simulink model "PardoSplitLabModel"  (R2024b)
settings: Solver=VariableStepAuto  StartTime=0.0  StopTime=10.0  RelTol=1e-3
libraries: simulink x8
settings Model: Creator=ferbe  LastModifiedBy=ferbe

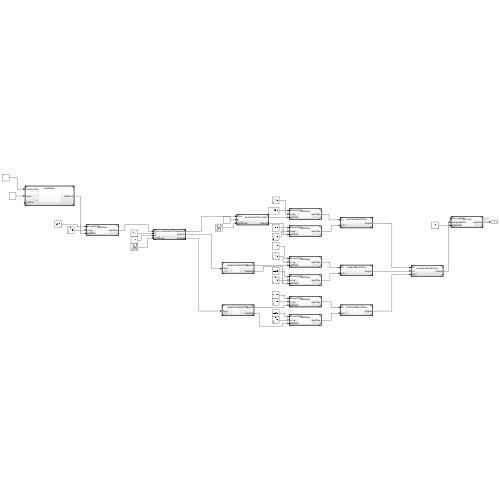
[thumbnail: Simulink's stored preview of the top-level diagram]
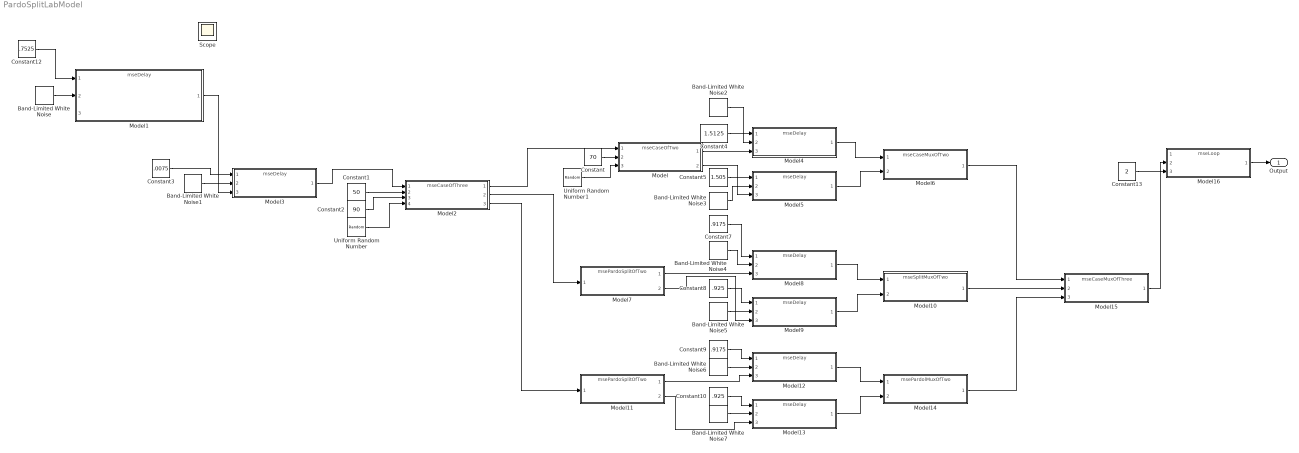
== system PardoSplitLabModel ==
  Band-Limited White Noise{,1..7} (8 alike) : simulink/Sources/Band-Limited White Noise  Cov=[0.1]  Ts=0.1  seed=[23341]
  Constant : Constant  Value=70
  Constant1 : Constant  Value=50
  Constant10 : Constant  Value=.925
  Constant12 : Constant  Value=.7525
  Constant13 : Constant  Value=2
  Constant2 : Constant  Value=90
  Constant3 : Constant  Value=.0075
  Constant4 : Constant  Value=1.5125
  Constant5 : Constant  Value=1.505
  Constant7 : Constant  Value=.9175
  Constant8 : Constant  Value=.925
  Constant9 : Constant  Value=.9175
  Model : ModelReference  ModelNameDialog=mseCaseOfTwo.slx  SimulationMode=Normal  ModelReferenceVersion=3.9
  Model{1,3..5,8..9,12..13} (8 alike) : ModelReference  ModelNameDialog=mseDelay.slx  SimulationMode=Normal  ModelReferenceVersion=3.3
  Model10 : ModelReference  ModelNameDialog=mseSplitMuxOfTwo.slx  SimulationMode=Normal  ModelReferenceVersion=3.2
  Model11 : ModelReference  ModelNameDialog=msePardoSplitOfTwo.slx  SimulationMode=Normal  ModelReferenceVersion=3.2
  Model14 : ModelReference  ModelNameDialog=msePardolMuxOfTwo.slx  SimulationMode=Normal  ModelReferenceVersion=3.3
  Model15 : ModelReference  ModelNameDialog=mseCaseMuxOfThree.slx  SimulationMode=Normal  ModelReferenceVersion=3.1
  Model16 : ModelReference  ModelNameDialog=mseLoop.slx  SimulationMode=Normal  ModelReferenceVersion=3.1
  Model2 : ModelReference  ModelNameDialog=mseCaseOfThree.slx  SimulationMode=Normal  ModelReferenceVersion=3.7
  Model6 : ModelReference  ModelNameDialog=mseCaseMuxOfTwo.slx  SimulationMode=Normal  ModelReferenceVersion=3.0
  Model7 : ModelReference  ModelNameDialog=msePardoSplitOfTwo.slx  SimulationMode=Normal  ModelReferenceVersion=3.2
  Uniform Random Number : UniformRandomNumber  Minimum=0  Maximum=100  SampleTime=0.1
  Uniform Random Number1 : UniformRandomNumber  Minimum=0  Maximum=100  SampleTime=0.1
  Output : Outport
  Scope : Scope
  wires:
  Band-Limited White Noise/1 -> Model1/2
  Uniform Random Number/1 -> Model2/4
  Constant1/1 -> Model2/2
  Constant2/1 -> Model2/3
  Model1/1 -> Model3/3
  Constant3/1 -> Model3/1
  Band-Limited White Noise1/1 -> Model3/2
  Model3/1 -> Model2/1
  Uniform Random Number1/1 -> Model/3
  Model2/1 -> Model/1
  Constant/1 -> Model/2
  Model/1 -> Model4/3
  Band-Limited White Noise2/1 -> Model4/2
  Constant4/1 -> Model4/1
  Model/2 -> Model5/3
  Constant5/1 -> Model5/1
  Band-Limited White Noise3/1 -> Model5/2
  Model4/1 -> Model6/1
  Model2/2 -> Model7/1
  Model7/1 -> Model8/3
  Constant7/1 -> Model8/1
  Band-Limited White Noise4/1 -> Model8/2
  Model7/2 -> Model9/3
  Constant8/1 -> Model9/1
  Band-Limited White Noise5/1 -> Model9/2
  Model8/1 -> Model10/1
  Model9/1 -> Model10/2
  Model2/3 -> Model11/1
  Model11/1 -> Model12/3
  Band-Limited White Noise6/1 -> Model12/2
  Constant9/1 -> Model12/1
  Constant10/1 -> Model13/1
  Model11/2 -> Model13/3
  Band-Limited White Noise7/1 -> Model13/2
  Model12/1 -> Model14/1
  Model13/1 -> Model14/2
  Model6/1 -> Model15/1
  Model10/1 -> Model15/2
  Model14/1 -> Model15/3
  Constant12/1 -> Model1/1
  Model16/1 -> Output/1
  Constant13/1 -> Model16/3
  Model15/1 -> Model16/2
  Model5/1 -> Model6/2
